simulink model "system"  (R2015b)
settings: Solver=FixedStepAuto  StartTime=0.0  StopTime=10.0  RelTol=1e-3
settings Model: Creator=Josef  LastModifiedBy=Josef
settings HardwareCC: ProdBitPerPointer=32  ProdWordSize=32  ProdHWDeviceType=Intel->x86-32 (Windows32)

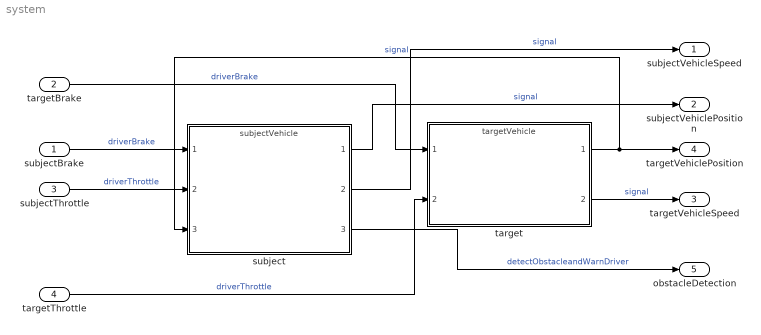
== system system ==
  subjectBrake : Inport
      settings: AttributesFormatString=driverBrake
  targetBrake : Inport  Port=2
      settings: AttributesFormatString=driverBrake
  subjectThrottle : Inport  Port=3
      settings: AttributesFormatString=driverThrottle
  targetThrottle : Inport  Port=4
      settings: AttributesFormatString=driverThrottle
  subject : ModelReference  ModelNameDialog=subjectVehicle  SimulationMode=Normal  ModelReferenceVersion=1.62  CopyOfModelName=subjectVehicle
  target : ModelReference  ModelNameDialog=targetVehicle  SimulationMode=Normal  ModelReferenceVersion=1.10  CopyOfModelName=subjectVehicle
  subjectVehicleSpeed : Outport
      settings: AttributesFormatString=signal
  subjectVehiclePosition : Outport  Port=2
      settings: AttributesFormatString=signal
  targetVehicleSpeed : Outport  Port=3
      settings: AttributesFormatString=signal
  targetVehiclePosition : Outport  Port=4
      settings: AttributesFormatString=signal
  obstacleDetection : Outport  Port=5
      settings: AttributesFormatString=detectObstacleandWarnDriver
  wires:
  target/1 -> subject/3, targetVehiclePosition/1  "signal"
  subjectBrake/1 -> subject/1  "driverBrake"
  targetBrake/1 -> target/1  "driverBrake"
  subjectThrottle/1 -> subject/2  "driverThrottle"
  targetThrottle/1 -> target/2  "driverThrottle"
  subject/1 -> subjectVehiclePosition/1  "signal"
  subject/2 -> subjectVehicleSpeed/1  "signal"
  target/2 -> targetVehicleSpeed/1  "signal"
  subject/3 -> obstacleDetection/1  "detectObstacleandWarnDriver"
